simulink model "sin_in"  (R2020a)
settings: Solver=ode4  StartTime=0.0  StopTime=10.0  RelTol=1e-3
settings Model: Creator=18423  LastModifiedBy=18423

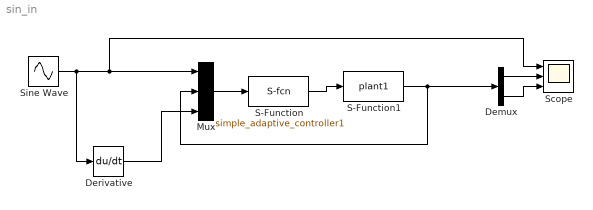
== system sin_in ==
  Demux : Demux  Outputs=2
  Derivative : Derivative
  Mux : Mux  Inputs=3
  S-Function : S-Function  FunctionName=simple_adaptive_controller1  SFunctionDeploymentMode=off  EnableBusSupport=off
  S-Function1 : S-Function  FunctionName=plant1  SFunctionDeploymentMode=off  EnableBusSupport=off
  Scope : Scope  NumInputPorts=3
  Sine Wave : Sin  SampleTime=0
  wires:
  Sine Wave/1 -> Scope/1, Mux/1, Derivative/1
  Derivative/1 -> Mux/3
  Mux/1 -> S-Function/1
  S-Function/1 -> S-Function1/1
  S-Function1/1 -> Demux/1, Mux/2
  Demux/2 -> Scope/3
  Demux/1 -> Scope/2
